simulink model "sampleModel12"  (R2021b)
settings: Solver=VariableStepAuto  StartTime=0.0  StopTime=10.0  RelTol=1e-3
undefined symbols (not defined in the file or in its folder): Newton, Raphson
libraries: simulink x19, slpidlib x1
settings Model: Creator=user  LastModifiedBy=user

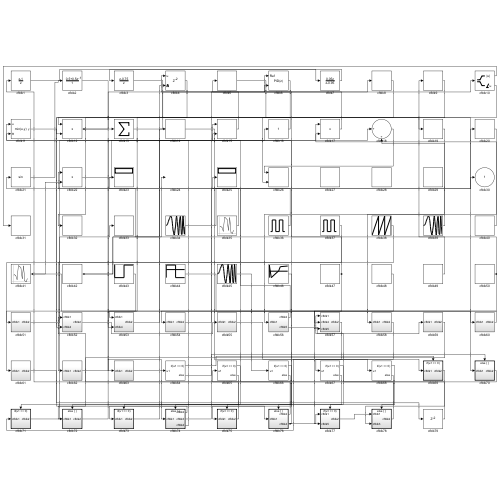
[thumbnail: Simulink's stored preview of the top-level diagram]
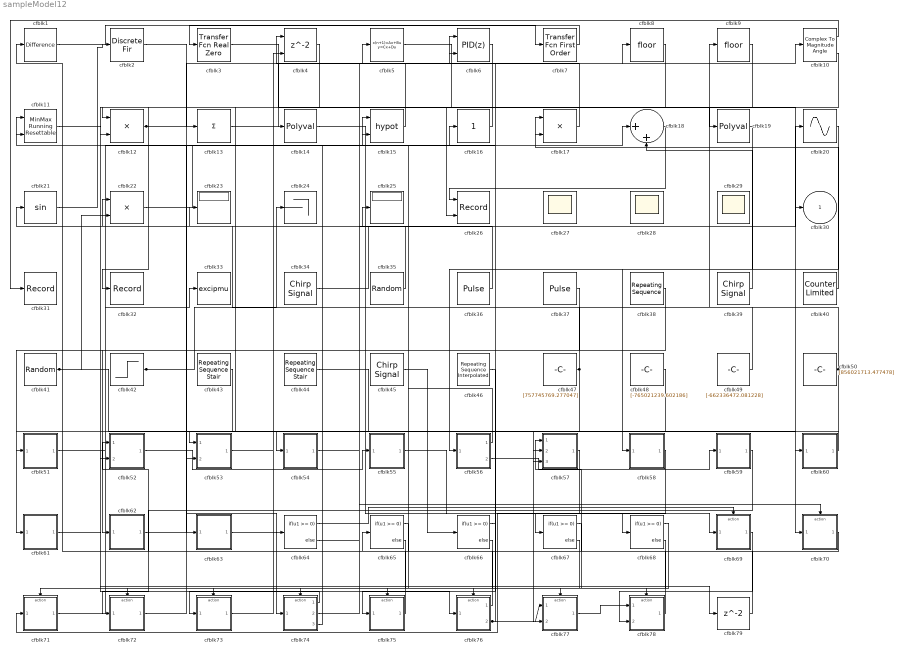
== system sampleModel12 ==
  cfblk1 : simulink/Discrete/Difference  ICPrevInput=0.0  OutMin=[]  OutMax=[]  OutDataTypeStr=Inherit: Inherit via back propagation  OutDataType=fixdt(1, 16)  OutScaling=2^-10  DoSatur=off
  cfblk10 : ComplexToMagnitudeAngle
  cfblk11 : simulink/Math Operations/MinMax Running Resettable  Function=min  vinit=0.0
  cfblk12 : Product
  cfblk13 : Sum  Inputs=+
  cfblk14 : Polyval  Coefs=[ +2.081618890e-019, -1.441693666e-014, +4.719686976e-010, -8.536869453e-006, +1.621573104e-001, -8.087801117e+001 ]
  cfblk15 : Math  Operator=hypot  SaturateOnIntegerOverflow=on
  cfblk16 : simulink/Math Operations/Slider Gain  gain=1  low=0  high=2
  cfblk17 : Product  Inputs=**
  cfblk18 : Sum  Inputs=|++
  cfblk19 : Polyval  Coefs=[ +2.081618890e-019, -1.441693666e-014, +4.719686976e-010, -8.536869453e-006, +1.621573104e-001, -8.087801117e+001 ]
  cfblk2 : DiscreteFir  SampleTime=1
  cfblk20 : Sin  TimeSource=Use external signal  SampleTime=0
  cfblk21 : Trigonometry
  cfblk22 : Product
  cfblk23 : Display
  cfblk24 : Terminator
  cfblk25 : Display
  cfblk26 : Record  FileSettingsInternal="{\"entries\":[{\"content\":{\"excelSettings\":{\"content\":{},\"type\":\"Streamout.ExcelSettings\"}},\"type\":\"Streamout.FileSettingStorage\",\"uuid\":\"1977bd0a-69a2-439d-8604-42371395555f\"}],\"packageUris\":[\"http://schema.mathworks.com/mf0/streamout_blocks/R2020a\"],\"version\":\"1.0\"}"  Layout=[1 1]  SignalsInternal="{\"entries\":[{\"content\":{\"signals\":[{\"content\":{\"blockPath\":[\"sampleModel12/cfblk26\"],\"channel\":[],\"dimensions\":[1],\"domain\":\"sampleModel12/cfblk26\",\"lineColor\":\"#a2142f\",\"plots\":[1],\"port\":1,\"sid\":[\"\"],\"signalID\":428,\"signalName\":\"cfblk18\"},\"type\":\"RecordBlkView.Signal\",\"uuid\":\"f3019e72-28ea-4570-a652-9e8685cbfb3c\"},{\"content\":{\"blockPath\":[\"sampleModel12/cfblk26\"],\"channel\":[],\"dimensions\":[1],\"domain\":\"sampleModel12/cfblk26\",\"lineColor\":\"#139fff\",\"plots\":[1],\"port\":2,\"sid\":[\"\"],\"signalID\":432,\"signalName\":\"cfblk10:2\"},\"type\":\"RecordBlkView.Signal\",\"uuid\":\"b0ef7f76-1df1-4dcb-8216-5290599b1a98\"}]},\"type\":\"RecordBlkView.InputSignals\",\"uuid\":\"a8e00ee3-3942-4fe2-8210-ac086d08e03d\"}],\"packageUris\":[\"http://schema.mathworks.com/mf0/streamout_blocks/R2020a\"],\"version\":\"1.0\"}"  VisualizationBindings="{\"xyplotplugin\":{\"info\":[{\"series\":[{\"bindingParametersList\":[{\"parameter\":\"X-Axis\",\"signalID\":428,\"signalName\":\"cfblk18\"},{\"parameter\":\"Y-Axis\",\"signalID\":432,\"signalName\":\"cfblk10:2\"}],\"seriesID\":23501}],\"subplotID\":1}]}}"  CompatibilityTag=XY
  cfblk27 : Scope
      settings: Floating=on
  cfblk28 : Scope
      settings: Floating=on
  cfblk29 : Scope
      settings: Floating=on
  cfblk3 : simulink/Discrete/Transfer Fcn Real Zero  ZeroZ=0.75  ICPrevInput=0.0  DoSatur=off
      settings: SourceProductBaseCode=SL
  cfblk31 : Record  FileSettingsInternal="{\"entries\":[{\"content\":{\"excelSettings\":{\"content\":{},\"type\":\"Streamout.ExcelSettings\"}},\"type\":\"Streamout.FileSettingStorage\",\"uuid\":\"da6b355c-110a-4d9d-8c85-11dfa9378df7\"}],\"packageUris\":[\"http://schema.mathworks.com/mf0/streamout_blocks/R2020a\"],\"version\":\"1.0\"}"  SignalsInternal="{\"entries\":[{\"content\":{\"signals\":[{\"content\":{\"blockPath\":[\"sampleModel12/cfblk31\"],\"channel\":[],\"dimensions\":[1],\"domain\":\"sampleModel12/cfblk31\",\"lineColor\":\"#edb120\",\"plots\":[1],\"port\":1,\"sid\":[\"\"],\"signalID\":436,\"signalName\":\"cfblk10:1\"},\"type\":\"RecordBlkView.Signal\",\"uuid\":\"ae69bb2e-39ac-490d-996f-805b6f004b7c\"}]},\"type\":\"RecordBlkView.InputSignals\",\"uuid\":\"de569a82-f94e-46d9-a337-50138a330fbc\"}],\"packageUris\":[\"http://schema.mathworks.com/mf0/streamout_blocks/R2020a\"],\"version\":\"1.0\"}"  VisualizationBindings="{\"sparklinesplugin\":{\"info\":[{\"bindingParametersList\":[],\"subplotID\":1}]}}"
  cfblk32 : Record  FileSettingsInternal="{\"entries\":[{\"content\":{\"excelSettings\":{\"content\":{},\"type\":\"Streamout.ExcelSettings\"}},\"type\":\"Streamout.FileSettingStorage\",\"uuid\":\"c9f7d570-c88d-4228-83d0-ca59f7ab4bdd\"}],\"packageUris\":[\"http://schema.mathworks.com/mf0/streamout_blocks/R2020a\"],\"version\":\"1.0\"}"  SignalsInternal="{\"entries\":[{\"content\":{\"signals\":[{\"content\":{\"blockPath\":[\"sampleModel12/cfblk32\"],\"channel\":[],\"dimensions\":[1],\"domain\":\"sampleModel12/cfblk32\",\"lineColor\":\"#7e2f8e\",\"plots\":[1],\"port\":1,\"sid\":[\"\"],\"signalID\":440,\"signalName\":\"cfblk8\"},\"type\":\"RecordBlkView.Signal\",\"uuid\":\"cca8ab52-b53e-444e-b4d0-924eaea725a7\"}]},\"type\":\"RecordBlkView.InputSignals\",\"uuid\":\"2acedad1-730a-4821-a658-abd68721b299\"}],\"packageUris\":[\"http://schema.mathworks.com/mf0/streamout_blocks/R2020a\"],\"version\":\"1.0\"}"  VisualizationBindings="{\"sparklinesplugin\":{\"info\":[{\"bindingParametersList\":[],\"subplotID\":1}]}}"
  cfblk33 : ToWorkspace  VariableName=excipmu  SaveFormat=Timeseries  SampleTime=-1
  cfblk34 : simulink/Sources/Chirp Signal  f1=[61556281.949611]  T=[-545379336.715425]  f2=[418969950.392962]
  cfblk35 : RandomNumber  Mean=[-70273.489359]  Variance=[65811.618122]  Seed=[633982548.000000]  SampleTime=0.1
  cfblk36 : DiscretePulseGenerator  PulseType=Time based  Amplitude=[-541387497.068457]  Period=[18222802.345042]  PulseWidth=5  PhaseDelay=[2.000000]
  cfblk37 : DiscretePulseGenerator  PulseType=Time based  Amplitude=[-700785816.762518]  Period=[20274740.571512]  PulseWidth=5  PhaseDelay=[9.000000]
  cfblk38 : simulink/Sources/Repeating Sequence  rep_seq_t=[0 2]  rep_seq_y=[-968183322.381030, 915028700.342366]
  cfblk39 : simulink/Sources/Chirp Signal  f1=[-948615429.259544]  T=[942221326.191418]  f2=[-404808646.483054]
  cfblk4 : Delay  ShowEnablePort=on  SampleTime=1
      settings: InputPortMap=u0,e6
  cfblk40 : simulink/Sources/Counter Limited  uplimit=[525.000000]  tsamp=-1
  cfblk41 : RandomNumber  Mean=[72467.842296]  Variance=[89640.490346]  Seed=[189010556.000000]  SampleTime=0.1
  cfblk42 : Step  Time=[33.000000]  Before=[882461875.746971]  After=[951414251.341264]  SampleTime=0
  cfblk43 : simulink/Sources/Repeating Sequence Stair  OutValues=[-784129493.964513, -642201543.955474]  tsamp=-1  OutMin=[]  OutMax=[]  OutDataTypeStr=double  OutputDataTypeScalingMode=double  OutDataType=fixdt(0,8)  ConRadixGroup=Best Precision: Vector-wise  OutScaling=2^-12
  cfblk44 : simulink/Sources/Repeating Sequence Stair  OutValues=[493102854.264072, -901062954.936100]  tsamp=-1  OutMin=[]  OutMax=[]  OutDataTypeStr=double  OutputDataTypeScalingMode=double  OutDataType=fixdt(0,8)  ConRadixGroup=Best Precision: Vector-wise  OutScaling=2^-12
  cfblk45 : simulink/Sources/Chirp Signal  f1=[-857430236.072932]  T=[-21748960.857344]  f2=[699787642.479273]
  cfblk46 : simulink/Sources/Repeating Sequence Interpolated  OutValues=[994082887.756000, -991214774.835649, 85214928.118158, 722696352.833129, 818278048.940125]  TimeValues=[0 0.1 0.5 0.6 1].'  LookUpMeth=Use Input Above  tsamp=0.01  OutMin=[]  OutMax=[]  OutDataTypeStr=double  OutputDataTypeScalingMode=double  OutDataType=fixdt(0,8)  OutScaling=2^-10
  cfblk47 : Constant  Value=[757745769.277047]  SampleTime=1
  cfblk48 : Constant  Value=[-765021239.602186]  SampleTime=1
  cfblk49 : Constant  Value=[-662336472.081228]  SampleTime=1
  cfblk5 : DiscreteStateSpace
  cfblk50 : Constant  Value=[856021713.477478]  SampleTime=1
  cfblk51 : Subsystem
  cfblk52 : Subsystem
  cfblk53 : Subsystem
  cfblk54 : Subsystem
  cfblk55 : Subsystem
  cfblk56 : Subsystem
  cfblk57 : Subsystem
  cfblk58 : Subsystem
  cfblk59 : Subsystem
  cfblk6 : slpidlib/PID Controller (2DOF)  Controller=PID  Form=Parallel  TimeDomain=Discrete-time  UseExternalTs=off  SampleTime=1  IntegratorMethod=Forward Euler  FilterMethod=Forward Euler  ControllerParametersSource=internal  P=1  I=1  D=0  UseFilter=on  N=100  b=1  c=1  TunerSelectOption=Transfer Function Based (PID Tuner App)  InitialConditionSource=internal  InitialConditionForIntegrator=0  InitialConditionForFilter=0  DifferentiatorICPrevScaledInput=0  ExternalReset=none  TrackingMode=off  Kt=1  LimitOutput=off  SatLimitsSource=internal  UpperSaturationLimit=inf  LowerSaturationLimit=-inf  LinearizeAsGain=off  AntiWindupMode=none  Kb=1  POutMin=[]  POutMax=[]  IOutMin=[]  IOutMax=[]  DOutMin=[]  DOutMax=[]  NOutMin=[]  NOutMax=[]  bOutMin=[]  bOutMax=[]  cOutMin=[]  cOutMax=[]  SumOutMin=[]  SumOutMax=[]  SaturationOutMin=[]  SaturationOutMax=[]  PParamMin=[]  PParamMax=[]  IParamMin=[]  IParamMax=[]  DParamMin=[]  DParamMax=[]  NParamMin=[]  NParamMax=[]  bParamMin=[]  bParamMax=[]  cParamMin=[]  cParamMax=[]  KbParamMin=[]  KbParamMax=[]  KtParamMin=[]  KtParamMax=[]  KbOutMin=[]  KbOutMax=[]  KtOutMin=[]  KtOutMax=[]  IntegratorOutMin=[]  IntegratorOutMax=[]  FilterOutMin=[]  FilterOutMax=[]  SumI1OutMin=[]  SumI1OutMax=[]  SumI2OutMin=[]  SumI2OutMax=[]  SumI3OutMin=[]  SumI3OutMax=[]  SumI4OutMin=[]  SumI4OutMax=[]  SumDOutMin=[]  SumDOutMax=[]  Sum1OutMin=[]  Sum1OutMax=[]  Sum2OutMin=[]  Sum2OutMax=[]  Sum3OutMin=[]  Sum3OutMax=[]  DifferentiatorOutMin=[]  DifferentiatorOutMax=[]  FilterDiffOutCoefMin=[]  FilterDiffOutCoefMax=[]  ReciprocalOutMin=[]  ReciprocalOutMax=[]  SumDenOutMin=[]  SumDenOutMax=[]  SumNumOutMin=[]  SumNumOutMax=[]  DivideOutMin=[]  DivideOutMax=[]  UdiffTsProdOutMin=[]  UdiffTsProdOutMax=[]  NTsProdOutMin=[]  NTsProdOutMax=[]  UintegralTsProdOutMin=[]  UintegralTsProdOutMax=[]  UngainTsProdOutMin=[]  UngainTsProdOutMax=[]  IntegratorContinuousStateAttributes=''  IntegratorStateMustResolveToSignalObject=off  IntegratorRTWStateStorageClass=Auto  FilterContinuousStateAttributes=''  FilterStateMustResolveToSignalObject=off  FilterRTWStateStorageClass=Auto  ParallelPVariant=InternalParameters  IdealPVariant=Disabled  IVariant=InternalParameters  DVariant=InternalParameters  bVariant=InternalParameters  cVariant=InternalParameters  IntegratorVariant=Discrete  SatVariant=Disabled  AWVariant=Passthrough  PCopyVariant=Disabled  TRVariant=Disabled  FdbkBlocksVariant=Forward  IdealPFdbkVariant=Disabled  SatFdbkVariant=Disabled  DerivativeFilterVariant=ForwardEulerFilter  NVariant=InternalParameters  NCopyVariant=Disabled  FilterICVariant=InternalICsFilter  IntegratorICVariant=InternalICs  ExternalResetVariant=Disabled  TRSumVariant=Passthrough  SumFdbkVariant=Disabled  SumVariant=Sum_PID  TsampFilterVariant=InternalTs  TsampNgainVariant=Passthrough  TsampIntegralVariant=Passthrough  ExternalSaturationOutDataTypeStr=Inherit: Same as second input
      settings: SourceProductBaseCode=SL
  cfblk60 : Subsystem
  cfblk61 : Subsystem
  cfblk62 : Subsystem
  cfblk63 : Subsystem
  cfblk{64..68} (5 alike) : If  IfExpression=u1 >= 0  SampleTime=1
  cfblk69 : Subsystem  TreatAsAtomicUnit=on
  cfblk7 : simulink/Discrete/Transfer Fcn First Order  PoleZ=0.95  ICPrevOutput=0.0  DoSatur=off
  cfblk70 : Subsystem  TreatAsAtomicUnit=on
  cfblk71 : Subsystem  TreatAsAtomicUnit=on
  cfblk72 : Subsystem  TreatAsAtomicUnit=on
  cfblk73 : Subsystem  TreatAsAtomicUnit=on
  cfblk74 : Subsystem  TreatAsAtomicUnit=on
  cfblk75 : Subsystem  TreatAsAtomicUnit=on
  cfblk76 : Subsystem  TreatAsAtomicUnit=on
  cfblk77 : Subsystem  TreatAsAtomicUnit=on
  cfblk78 : Subsystem  TreatAsAtomicUnit=on
  cfblk79 : Delay  SampleTime=1
  cfblk8 : Rounding
  cfblk9 : Rounding
  cfblk30 : Outport
  wires:
  cfblk71/1(cfblk2) -> cfblk17/1
  cfblk20/1 -> cfblk56/1(cfblk1)
  cfblk40/1 -> cfblk17/2
  cfblk74/1(cfblk2) -> cfblk73/1(cfblk1)
  cfblk51/1(cfblk2) -> cfblk33/1
  cfblk2/1 -> cfblk63/1(cfblk1)
  cfblk4/1 -> cfblk53/1(cfblk1)
  cfblk42/1 -> cfblk24/1, cfblk4/2
  cfblk7/1 -> cfblk3/1
  cfblk46/1 -> cfblk75/1(cfblk1)
  cfblk36/1 -> cfblk21/1
  cfblk13/1 -> cfblk10/1
  cfblk35/1 -> cfblk22/1
  cfblk45/1 -> cfblk66/1
  cfblk10/1 -> cfblk31/1
  cfblk57/1(cfblk2) -> cfblk71/1(cfblk1)
  cfblk55/1(cfblk2) -> cfblk68/1
  cfblk77/1(cfblk2) -> cfblk78/1(cfblk1)
  cfblk53/1(cfblk2) -> cfblk14/1
  cfblk43/1 -> cfblk61/1(cfblk1)
  cfblk14/1 -> cfblk69/1(cfblk1)
  cfblk1/1 -> cfblk7/1
  cfblk49/1 -> cfblk9/1
  cfblk37/1 -> cfblk51/1(cfblk1)
  cfblk3/1 -> cfblk19/1
  cfblk58/1(cfblk2) -> cfblk67/1
  cfblk18/1 -> cfblk26/1
  cfblk70/1(cfblk2) -> cfblk65/1
  cfblk44/1 -> cfblk70/1(cfblk1)
  cfblk69/1(cfblk2) -> cfblk78/2(cfblk3)
  cfblk17/1 -> cfblk5/1
  cfblk38/1 -> cfblk62/1(cfblk1)
  cfblk76/1(cfblk2) -> cfblk25/1
  cfblk61/1(cfblk2) -> cfblk76/1(cfblk1)
  cfblk75/1(cfblk2) -> cfblk52/1(cfblk1)
  cfblk10/2 -> cfblk26/2
  cfblk22/1 -> cfblk16/1
  cfblk6/1 -> cfblk52/2(cfblk4)
  cfblk15/1 -> cfblk4/1
  cfblk63/1(cfblk2) -> cfblk74/1(cfblk1)
  cfblk78/1(cfblk2) -> cfblk57/1(cfblk1)
  cfblk76/2(cfblk4) -> cfblk77/1(cfblk1), cfblk11/2
  cfblk74/2(cfblk3) -> cfblk8/1
  cfblk8/1 -> cfblk32/1
  cfblk72/1(cfblk2) -> cfblk15/1
  cfblk5/1 -> cfblk60/1(cfblk1)
  cfblk60/1(cfblk2) -> cfblk54/1(cfblk1)
  cfblk16/1 -> cfblk12/1
  cfblk12/1 -> cfblk13/1, cfblk6/2
  cfblk47/1 -> cfblk23/1, cfblk57/3(cfblk5)
  cfblk73/1(cfblk2) -> cfblk18/1
  cfblk34/1 -> cfblk20/1
  cfblk21/1 -> cfblk2/1
  cfblk9/1 -> cfblk12/2
  cfblk19/1 -> cfblk58/1(cfblk1)
  cfblk52/1(cfblk2) -> cfblk55/1(cfblk1)
  cfblk56/1(cfblk2) -> cfblk15/2
  cfblk39/1 -> cfblk18/2
  cfblk48/1 -> cfblk53/2(cfblk4)
  cfblk59/1(cfblk2) -> cfblk72/1(cfblk1)
  cfblk62/1(cfblk2) -> cfblk64/1
  cfblk56/2(cfblk5) -> cfblk59/1(cfblk1)
  cfblk54/1(cfblk2) -> cfblk30/1
  cfblk50/1 -> cfblk6/1, cfblk57/2(cfblk4)
  cfblk41/1 -> cfblk77/2(cfblk5), cfblk22/2
  cfblk74/3(cfblk4) -> cfblk11/1
  cfblk64/1 -> cfblk69/Action
  cfblk64/2 -> cfblk70/Action
  cfblk65/1 -> cfblk71/Action
  cfblk65/2 -> cfblk72/Action
  cfblk66/1 -> cfblk73/Action
  cfblk66/2 -> cfblk74/Action
  cfblk67/1 -> cfblk75/Action
  cfblk67/2 -> cfblk76/Action
  cfblk68/1 -> cfblk77/Action
  cfblk68/2 -> cfblk78/Action
  cfblk11/1 -> cfblk79/1
  cfblk79/1 -> cfblk1/1

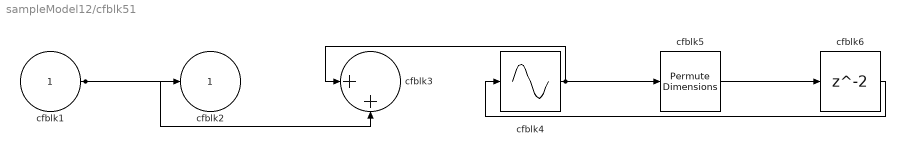
== system sampleModel12/cfblk51 ==
  cfblk1 : Inport
  cfblk3 : Sum  Inputs=|++
  cfblk4 : Sin  TimeSource=Use external signal  SampleTime=0
  cfblk5 : PermuteDimensions
  cfblk6 : Delay  SampleTime=1
  cfblk2 : Outport
  wires:
  cfblk1/1 -> cfblk2/1, cfblk3/2
  cfblk4/1 -> cfblk5/1, cfblk3/1
  cfblk5/1 -> cfblk6/1
  cfblk6/1 -> cfblk4/1

== system sampleModel12/cfblk52 ==
  cfblk1 : Inport
  cfblk4 : Inport  Port=2
  cfblk3 : simulink/Discrete/Transfer Fcn First Order  PoleZ=0.95  ICPrevOutput=0.0  DoSatur=off
  cfblk2 : Outport
  wires:
  cfblk1/1 -> cfblk3/1
  cfblk4/1 -> cfblk2/1

== system sampleModel12/cfblk53 ==
  cfblk1 : Inport
  cfblk4 : Inport  Port=2
  cfblk3 : simulink/Discrete/Transfer Fcn First Order  PoleZ=0.95  ICPrevOutput=0.0  DoSatur=off
  cfblk2 : Outport
  wires:
  cfblk4/1 -> cfblk3/1
  cfblk1/1 -> cfblk2/1

== system sampleModel12/cfblk54 ==
  cfblk1 : Inport
  cfblk3 : UnaryMinus
  cfblk4 : Sqrt  Operator=rSqrt  AlgorithmType=Newton-Raphson  SaturateOnIntegerOverflow=on
  cfblk2 : Outport
  wires:
  cfblk4/1 -> cfblk3/1
  cfblk1/1 -> cfblk4/1
  cfblk3/1 -> cfblk2/1

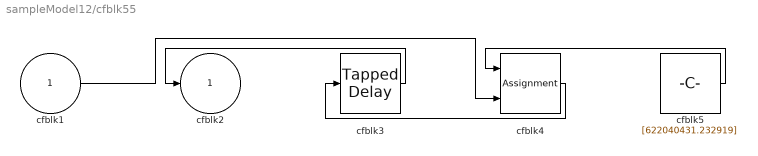
== system sampleModel12/cfblk55 ==
  cfblk1 : Inport
  cfblk3 : simulink/Discrete/Tapped Delay  vinit=0.0  samptime=-1  NumDelays=1  DelayOrder=Oldest  includeCurrent=off
  cfblk4 : Assignment  DiagnosticForDimensions=Warning  IndexOptions=Index vector (dialog)  Indices=1  OutputSizes=1
  cfblk5 : Constant  Value=[622040431.232919]  SampleTime=1
  cfblk2 : Outport
  wires:
  cfblk5/1 -> cfblk4/1
  cfblk3/1 -> cfblk2/1
  cfblk4/1 -> cfblk3/1
  cfblk1/1 -> cfblk4/2

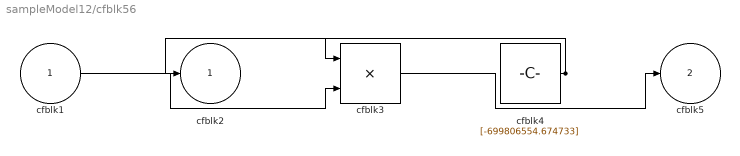
== system sampleModel12/cfblk56 ==
  cfblk1 : Inport
  cfblk3 : Product  Inputs=**
  cfblk4 : Constant  Value=[-699806554.674733]  SampleTime=1
  cfblk2 : Outport
  cfblk5 : Outport  Port=2
  wires:
  cfblk4/1 -> cfblk3/1, cfblk2/1
  cfblk3/1 -> cfblk5/1
  cfblk1/1 -> cfblk3/2

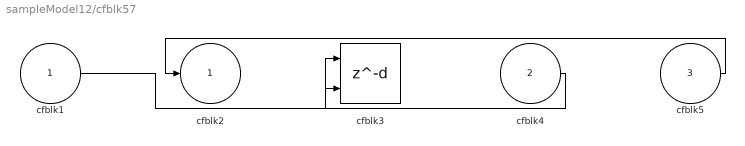
== system sampleModel12/cfblk57 ==
  cfblk1 : Inport
  cfblk4 : Inport  Port=2
  cfblk5 : Inport  Port=3
  cfblk3 : Delay  DelayLengthSource=Input port  SampleTime=1
      settings: InputPortMap=u0,p1
  cfblk2 : Outport
  wires:
  cfblk5/1 -> cfblk2/1
  cfblk1/1 -> cfblk3/1
  cfblk4/1 -> cfblk3/2

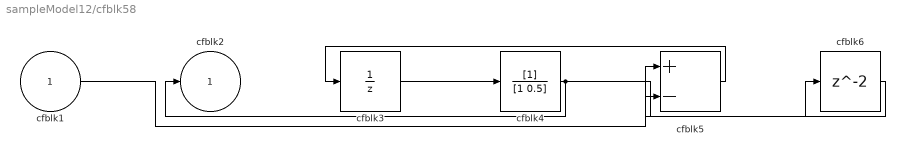
== system sampleModel12/cfblk58 ==
  cfblk1 : Inport
  cfblk3 : UnitDelay  HasFrameUpgradeWarning=on
  cfblk4 : DiscreteFilter  SampleTime=1
  cfblk5 : Sum  Inputs=+-
  cfblk6 : Delay  SampleTime=1
  cfblk2 : Outport
  wires:
  cfblk5/1 -> cfblk3/1
  cfblk4/1 -> cfblk2/1, cfblk6/1
  cfblk3/1 -> cfblk4/1
  cfblk1/1 -> cfblk5/1
  cfblk6/1 -> cfblk5/2

== system sampleModel12/cfblk59 ==
  cfblk1 : Inport
  cfblk3 : Abs
  cfblk2 : Outport
  wires:
  cfblk1/1 -> cfblk2/1, cfblk3/1

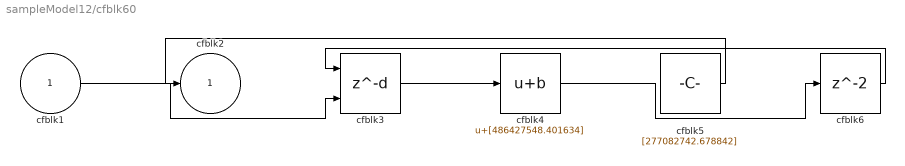
== system sampleModel12/cfblk60 ==
  cfblk1 : Inport
  cfblk3 : Delay  DelayLengthSource=Input port  SampleTime=1
      settings: InputPortMap=u0,p1
  cfblk4 : Bias  Bias=[486427548.401634]
  cfblk5 : Constant  Value=[277082742.678842]  SampleTime=1
  cfblk6 : Delay  SampleTime=1
  cfblk2 : Outport
  wires:
  cfblk1/1 -> cfblk3/2
  cfblk5/1 -> cfblk2/1
  cfblk3/1 -> cfblk4/1
  cfblk4/1 -> cfblk6/1
  cfblk6/1 -> cfblk3/1

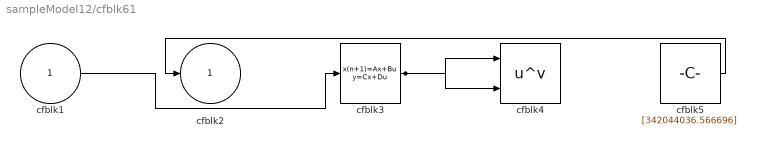
== system sampleModel12/cfblk61 ==
  cfblk1 : Inport
  cfblk3 : DiscreteStateSpace
  cfblk4 : Math  Operator=pow  SaturateOnIntegerOverflow=on
  cfblk5 : Constant  Value=[342044036.566696]  SampleTime=1
  cfblk2 : Outport
  wires:
  cfblk5/1 -> cfblk2/1
  cfblk3/1 -> cfblk4/1, cfblk4/2
  cfblk1/1 -> cfblk3/1

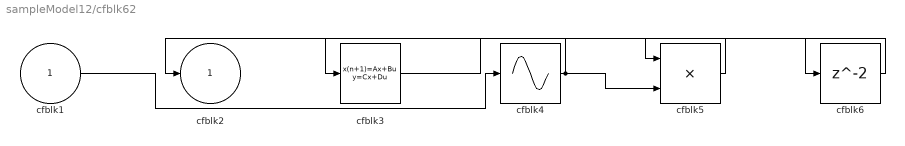
== system sampleModel12/cfblk62 ==
  cfblk1 : Inport
  cfblk3 : DiscreteStateSpace
  cfblk4 : Sin  TimeSource=Use external signal  SampleTime=0
  cfblk5 : Product
  cfblk6 : Delay  SampleTime=1
  cfblk2 : Outport
  wires:
  cfblk5/1 -> cfblk3/1
  cfblk4/1 -> cfblk2/1, cfblk5/2
  cfblk1/1 -> cfblk4/1
  cfblk3/1 -> cfblk6/1
  cfblk6/1 -> cfblk5/1

== system sampleModel12/cfblk63 ==
  cfblk1 : Inport
  cfblk3 : simulink/Discrete/Difference  ICPrevInput=0.0  OutMin=[]  OutMax=[]  OutDataTypeStr=Inherit: Inherit via back propagation  OutDataType=fixdt(1, 16)  OutScaling=2^-10  DoSatur=off
  cfblk4 : Constant  Value=[-908683353.045234]  SampleTime=1
  cfblk2 : Outport
  wires:
  cfblk1/1 -> cfblk3/1
  cfblk3/1 -> cfblk2/1

== system sampleModel12/cfblk69 ==
  cfblk1 : Inport
  Action Port : ActionPort  ActionPortLabel=if(u1 >= 0)
  cfblk3 : Constant  Value=[946689413.441740]  SampleTime=1
  cfblk2 : Outport
  wires:
  cfblk1/1 -> cfblk2/1

== system sampleModel12/cfblk70 ==
  cfblk1 : Inport
  Action Port : ActionPort  ActionPortLabel=else
  cfblk3 : Sum  Inputs=--
  cfblk2 : Outport
  wires:
  cfblk3/1 -> cfblk2/1
  cfblk1/1 -> cfblk3/1, cfblk3/2

== system sampleModel12/cfblk71 ==
  cfblk1 : Inport
  Action Port : ActionPort  ActionPortLabel=if(u1 >= 0)
  cfblk3 : Product  Inputs=*
  cfblk2 : Outport
  wires:
  cfblk3/1 -> cfblk2/1
  cfblk1/1 -> cfblk3/1

== system sampleModel12/cfblk72 ==
  cfblk1 : Inport
  Action Port : ActionPort  ActionPortLabel=else
  cfblk3 : Sqrt  Operator=rSqrt  AlgorithmType=Newton-Raphson  SaturateOnIntegerOverflow=on
  cfblk2 : Outport
  wires:
  cfblk1/1 -> cfblk3/1
  cfblk3/1 -> cfblk2/1

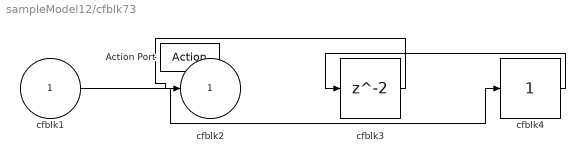
== system sampleModel12/cfblk73 ==
  cfblk1 : Inport
  Action Port : ActionPort  ActionPortLabel=if(u1 >= 0)
  cfblk3 : Delay
  cfblk4 : simulink/Math Operations/Slider Gain  gain=1  low=0  high=2
  cfblk2 : Outport
  wires:
  cfblk1/1 -> cfblk4/1
  cfblk3/1 -> cfblk2/1
  cfblk4/1 -> cfblk3/1

== system sampleModel12/cfblk74 ==
  cfblk1 : Inport
  Action Port : ActionPort  ActionPortLabel=else
  cfblk2 : Outport
  cfblk3 : Outport  Port=2
  cfblk4 : Outport  Port=3
  wires:
  cfblk1/1 -> cfblk2/1, cfblk3/1, cfblk4/1

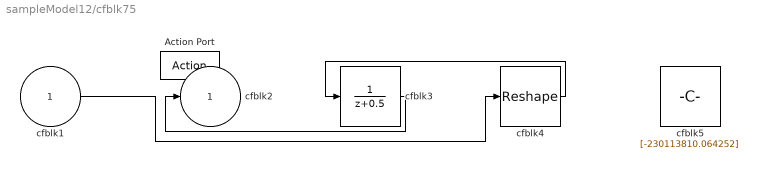
== system sampleModel12/cfblk75 ==
  cfblk1 : Inport
  Action Port : ActionPort  ActionPortLabel=if(u1 >= 0)
  cfblk3 : DiscreteTransferFcn
  cfblk4 : Reshape
  cfblk5 : Constant  Value=[-230113810.064252]  SampleTime=1
  cfblk2 : Outport
  wires:
  cfblk4/1 -> cfblk3/1
  cfblk3/1 -> cfblk2/1
  cfblk1/1 -> cfblk4/1

== system sampleModel12/cfblk76 ==
  cfblk1 : Inport
  Action Port : ActionPort  ActionPortLabel=else
  cfblk3 : Product  Inputs=**
  cfblk2 : Outport
  cfblk4 : Outport  Port=2
  wires:
  cfblk1/1 -> cfblk3/1, cfblk3/2
  cfblk3/1 -> cfblk2/1, cfblk4/1

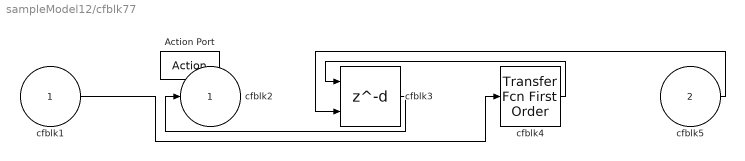
== system sampleModel12/cfblk77 ==
  cfblk1 : Inport
  cfblk5 : Inport  Port=2
  Action Port : ActionPort  ActionPortLabel=if(u1 >= 0)
  cfblk3 : Delay  DelayLengthSource=Input port
      settings: InputPortMap=u0,p1
  cfblk4 : simulink/Discrete/Transfer Fcn First Order  PoleZ=0.95  ICPrevOutput=0.0  DoSatur=off
  cfblk2 : Outport
  wires:
  cfblk3/1 -> cfblk2/1
  cfblk1/1 -> cfblk4/1
  cfblk4/1 -> cfblk3/1
  cfblk5/1 -> cfblk3/2

== system sampleModel12/cfblk78 ==
  cfblk1 : Inport
  cfblk3 : Inport  Port=2
  Action Port : ActionPort  ActionPortLabel=else
  cfblk2 : Outport
  wires:
  cfblk1/1 -> cfblk2/1
